simulink model "BaseEngineController_LS_112"  (Simulink 7.7)
settings: Solver=FixedStepDiscrete  StartTime=0.0  StopTime=10.0  RelTol=1e-3
PreLoadFcn:
  | try, eval([bdroot '_setup']); catch, eval('model_setup', ''); end
InitFcn:
  | try, eval([bdroot '_setup']); catch, eval('model_setup', ''); end
undefined symbols (not defined in the file): ECM, H1, H2, High, motohawk_build_version, motohawk_trunc_name, motohawk_vardec_config_group, motohawk_vardec_path, True, xD
libraries: MotoHawk_lib x1417, motohawk_control_primitives_lib x183, motohawk_engine_lib x32, simulink x21, motohawk_annotations_lib x9, AutoDoc_lib x8, simulink_extras x4, motohawk_ccp_examples_lib x1, motohawk_control_primitives_motoshare_lib x1
(part 10 of 27)

== system BaseEngineController_LS_112/Foreground/Outputs/AEM Infinity Dash/Dash Message Boost ==
  Data : Inport
  Bus Selector : BusSelector  OutputSignals=Sensors.Raw.NonLinearSensors.CAT
  Constant : Constant  Value=0
  Constant1 : Constant  Value=0
  Send CAN Messages : MotoHawk_lib/CAN Blocks/Send CAN Messages  bus=-2  nam='CAN_1'  msgl=CANTx_AEM_DASH_Boost  pace=5  labelwires=off
  motohawk_data_read : MotoHawk_lib/Data Storage Blocks/motohawk_data_read  source=Lookup By Name  structure=Scalar  operation=Read scalar from location by index  sz_vec=4  sz_row=2  sz_col=3  typ=double  nam='BoostControlTarget'  checkNull=on  struct_inst_name='MyData'  struct_nam='MyStruct'
  motohawk_data_read1 : MotoHawk_lib/Data Storage Blocks/motohawk_data_read  source=Lookup By Name  structure=Scalar  operation=Read scalar from location by index  sz_vec=4  sz_row=2  sz_col=3  typ=uint8  nam='BoostControlDutyCycleFF'  checkNull=on  struct_inst_name='MyData'  struct_nam='MyStruct'
  motohawk_data_read2 : MotoHawk_lib/Data Storage Blocks/motohawk_data_read  source=Lookup By Name  structure=Scalar  operation=Read scalar from location by index  sz_vec=4  sz_row=2  sz_col=3  typ=double  nam='BoostControlPID'  checkNull=on  struct_inst_name='MyData'  struct_nam='MyStruct'
  wires:
  Data/1 -> Bus Selector/1
  motohawk_data_read/1 -> Send CAN Messages/1
  Constant/1 -> Send CAN Messages/2
  motohawk_data_read1/1 -> Send CAN Messages/3
  motohawk_data_read2/1 -> Send CAN Messages/4
  Bus Selector/1 -> Send CAN Messages/5  "<CAT>"
  Constant1/1 -> Send CAN Messages/6

== system BaseEngineController_LS_112/Foreground/Outputs/AEM Infinity Dash/Dash Message DBW ==
  Data : Inport
  Bus Selector : BusSelector  OutputSignals=Sensors.RawProcessed.APPPcnt,Sensors.RawProcessed.ETCRequest,Sensors.Raw.PotSensors.TPS1,Sensors.Raw.PotSensors.TPS2
  Constant{1..8} (8 alike) : Constant  Value=0
  First Order Low Pass (Tunable) : motohawk_control_primitives_lib/First Order Low Pass (Tunable)  SystemSampleTime=-1  nam='ETCReq_Filt'  samp_time=-1  group=motohawk_vardec_path(gcb)
  First Order Low Pass (Tunable)1 : motohawk_control_primitives_lib/First Order Low Pass (Tunable)  SystemSampleTime=-1  nam='APP_Filt'  samp_time=-1  group=motohawk_vardec_path(gcb)
  Logical Operator{1..5} (5 alike) : Logic  Operator=OR  AllPortsSameDT=off  OutDataTypeStr=boolean
  Send CAN Messages : MotoHawk_lib/CAN Blocks/Send CAN Messages  bus=-2  nam='CAN_1'  msgl=CANTx_AEM_DASH_DBW  pace=5  labelwires=off
  motohawk_data_read1 : MotoHawk_lib/Data Storage Blocks/motohawk_data_read  source=Lookup By Name  structure=Scalar  operation=Read scalar from location by index  sz_vec=4  sz_row=2  sz_col=3  typ=boolean  nam='ETB_Curr_Flt'  checkNull=on  struct_inst_name='MyData'  struct_nam='MyStruct'
  motohawk_fault_status1 : MotoHawk_lib/Fault Management Blocks/motohawk_fault_status  source=Lookup By Name  nam='APP1RangeHigh'  status=Active
  motohawk_fault_status10 : MotoHawk_lib/Fault Management Blocks/motohawk_fault_status  source=Lookup By Name  nam='APP1RangeLow'  status=Active
  motohawk_fault_status11 : MotoHawk_lib/Fault Management Blocks/motohawk_fault_status  source=Lookup By Name  nam='TPS2RangeLow'  status=Active
  motohawk_fault_status12 : MotoHawk_lib/Fault Management Blocks/motohawk_fault_status  source=Lookup By Name  nam='TPS_Sensors_Conflict'  status=Active
  motohawk_fault_status2 : MotoHawk_lib/Fault Management Blocks/motohawk_fault_status  source=Lookup By Name  nam='APP2RangeHigh'  status=Active
  motohawk_fault_status3 : MotoHawk_lib/Fault Management Blocks/motohawk_fault_status  source=Lookup By Name  nam='APP2RangeLow'  status=Active
  motohawk_fault_status4 : MotoHawk_lib/Fault Management Blocks/motohawk_fault_status  source=Lookup By Name  nam='TPS1RangeHigh'  status=Active
  motohawk_fault_status5 : MotoHawk_lib/Fault Management Blocks/motohawk_fault_status  source=Lookup By Name  nam='ETC_Sticking'  status=Active
  motohawk_fault_status6 : MotoHawk_lib/Fault Management Blocks/motohawk_fault_status  source=Lookup By Name  nam='ETC_Open_Fault'  status=Active
  motohawk_fault_status7 : MotoHawk_lib/Fault Management Blocks/motohawk_fault_status  source=Lookup By Name  nam='TPS1RangeLow'  status=Active
  motohawk_fault_status8 : MotoHawk_lib/Fault Management Blocks/motohawk_fault_status  source=Lookup By Name  nam='TPS2RangeHigh'  status=Active
  motohawk_fault_status9 : MotoHawk_lib/Fault Management Blocks/motohawk_fault_status  source=Lookup By Name  nam='APP_Sensors_Conflict'  status=Active
  wires:
  Data/1 -> Bus Selector/1
  Bus Selector/1 -> First Order Low Pass (Tunable)1/1  "<APPPcnt>"
  Bus Selector/2 -> First Order Low Pass (Tunable)/1  "<ETCRequest>"
  Bus Selector/3 -> Send CAN Messages/3  "<TPS1>"
  Bus Selector/4 -> Send CAN Messages/4  "<TPS2>"
  motohawk_fault_status9/1 -> Send CAN Messages/5
  motohawk_fault_status10/1 -> Logical Operator3/1
  motohawk_fault_status1/1 -> Logical Operator3/2
  Logical Operator3/1 -> Send CAN Messages/6
  motohawk_fault_status3/1 -> Logical Operator1/1
  motohawk_fault_status2/1 -> Logical Operator1/2
  Logical Operator1/1 -> Send CAN Messages/7
  Constant1/1 -> Send CAN Messages/8
  Constant2/1 -> Send CAN Messages/20
  Constant3/1 -> Send CAN Messages/19
  Constant4/1 -> Send CAN Messages/18
  Constant5/1 -> Send CAN Messages/17
  Constant6/1 -> Send CAN Messages/16
  Constant7/1 -> Send CAN Messages/15
  motohawk_fault_status5/1 -> Logical Operator2/2
  motohawk_fault_status6/1 -> Logical Operator2/1
  Logical Operator2/1 -> Send CAN Messages/9
  motohawk_fault_status4/1 -> Logical Operator4/2
  motohawk_fault_status7/1 -> Logical Operator4/1
  Logical Operator4/1 -> Send CAN Messages/10
  motohawk_fault_status8/1 -> Logical Operator5/2
  motohawk_fault_status11/1 -> Logical Operator5/1
  Logical Operator5/1 -> Send CAN Messages/11
  motohawk_fault_status12/1 -> Send CAN Messages/14
  motohawk_data_read1/1 -> Send CAN Messages/13
  Constant8/1 -> Send CAN Messages/12
  First Order Low Pass (Tunable)1/1 -> Send CAN Messages/1
  First Order Low Pass (Tunable)/1 -> Send CAN Messages/2

== system BaseEngineController_LS_112/Foreground/Outputs/Coil Control/Coil Enable Manager ==
  CompareTo : motohawk_control_primitives_lib/CompareTo  SystemSampleTime=-1  op===  val=1
  EST Enable TDC Counter : Subsystem  TreatAsAtomicUnit=on
  Logical Operator1 : Logic  Operator=NOT  AllPortsSameDT=off  OutDataTypeStr=boolean
  Logical Operator2 : Logic  Inputs=6  AllPortsSameDT=off  OutDataTypeStr=boolean
  Logical Operator3 : Logic  Operator=NOT  AllPortsSameDT=off  OutDataTypeStr=boolean
  Logical Operator4 : Logic  Operator=NOT  AllPortsSameDT=off  OutDataTypeStr=boolean
  Mux : Mux  Inputs=8
  motohawk_calibration1 : MotoHawk_lib/Calibration & Probing Blocks/motohawk_calibration  nam='SparkEnableCyl5'  val=true  storage=Calibration  show_more=on  name_source=Use Parameter  data_type=Inherit via back propagation  read_level=1  write_level=1  ovr_cals=on  view_as=Enumeration  enum_struct={'Disabled', 'Enabled'}  vector_style=Wide Row  use_help_units=on  help='Disable spark to particular cylinder.'  units='boolean'  use_header_enum=off  row_header_enum={}  col_header_enum={}  use_min_max=off  min_val=-inf  max_val=inf  use_precision=off  precision=''  gain=1  offset=0  exp=1  use_mototune_group=on  mototune_group=motohawk_vardec_path(gcb)
  motohawk_calibration3 : MotoHawk_lib/Calibration & Probing Blocks/motohawk_calibration  nam='SparkEnableCyl1'  val=true  storage=Calibration  show_more=on  name_source=Use Parameter  data_type=Inherit via back propagation  read_level=1  write_level=1  ovr_cals=on  view_as=Enumeration  enum_struct={'Disabled', 'Enabled'}  vector_style=Wide Row  use_help_units=on  help='Disable spark to particular cylinder.'  units='boolean'  use_header_enum=off  row_header_enum={}  col_header_enum={}  use_min_max=off  min_val=-inf  max_val=inf  use_precision=off  precision=''  gain=1  offset=0  exp=1  use_mototune_group=on  mototune_group=motohawk_vardec_path(gcb)
  motohawk_calibration4 : MotoHawk_lib/Calibration & Probing Blocks/motohawk_calibration  nam='SparkEnableCyl2'  val=true  storage=Calibration  show_more=on  name_source=Use Parameter  data_type=Inherit via back propagation  read_level=1  write_level=1  ovr_cals=on  view_as=Enumeration  enum_struct={'Disabled', 'Enabled'}  vector_style=Wide Row  use_help_units=on  help='Disable spark to particular cylinder.'  units='boolean'  use_header_enum=off  row_header_enum={}  col_header_enum={}  use_min_max=off  min_val=-inf  max_val=inf  use_precision=off  precision=''  gain=1  offset=0  exp=1  use_mototune_group=on  mototune_group=motohawk_vardec_path(gcb)
  motohawk_calibration5 : MotoHawk_lib/Calibration & Probing Blocks/motohawk_calibration  nam='SparkEnableCyl3'  val=true  storage=Calibration  show_more=on  name_source=Use Parameter  data_type=Inherit via back propagation  read_level=1  write_level=1  ovr_cals=on  view_as=Enumeration  enum_struct={'Disabled', 'Enabled'}  vector_style=Wide Row  use_help_units=on  help='Disable spark to particular cylinder.'  units='boolean'  use_header_enum=off  row_header_enum={}  col_header_enum={}  use_min_max=off  min_val=-inf  max_val=inf  use_precision=off  precision=''  gain=1  offset=0  exp=1  use_mototune_group=on  mototune_group=motohawk_vardec_path(gcb)
  motohawk_calibration6 : MotoHawk_lib/Calibration & Probing Blocks/motohawk_calibration  nam='SparkEnableCyl4'  val=true  storage=Calibration  show_more=on  name_source=Use Parameter  data_type=Inherit via back propagation  read_level=1  write_level=1  ovr_cals=on  view_as=Enumeration  enum_struct={'Disabled', 'Enabled'}  vector_style=Wide Row  use_help_units=on  help='Disable spark to particular cylinder.'  units='boolean'  use_header_enum=off  row_header_enum={}  col_header_enum={}  use_min_max=off  min_val=-inf  max_val=inf  use_precision=off  precision=''  gain=1  offset=0  exp=1  use_mototune_group=on  mototune_group=motohawk_vardec_path(gcb)
  motohawk_calibration7 : MotoHawk_lib/Calibration & Probing Blocks/motohawk_calibration  nam='SparkEnableCyl6'  val=true  storage=Calibration  show_more=on  name_source=Use Parameter  data_type=Inherit via back propagation  read_level=1  write_level=1  ovr_cals=on  view_as=Enumeration  enum_struct={'Disabled', 'Enabled'}  vector_style=Wide Row  use_help_units=on  help='Disable spark to particular cylinder.'  units='boolean'  use_header_enum=off  row_header_enum={}  col_header_enum={}  use_min_max=off  min_val=-inf  max_val=inf  use_precision=off  precision=''  gain=1  offset=0  exp=1  use_mototune_group=on  mototune_group=motohawk_vardec_path(gcb)
  motohawk_calibration8 : MotoHawk_lib/Calibration & Probing Blocks/motohawk_calibration  nam='SparkEnableCyl7'  val=true  storage=Calibration  show_more=on  name_source=Use Parameter  data_type=Inherit via back propagation  read_level=1  write_level=1  ovr_cals=on  view_as=Enumeration  enum_struct={'Disabled', 'Enabled'}  vector_style=Wide Row  use_help_units=on  help='Disable spark to particular cylinder.'  units='boolean'  use_header_enum=off  row_header_enum={}  col_header_enum={}  use_min_max=off  min_val=-inf  max_val=inf  use_precision=off  precision=''  gain=1  offset=0  exp=1  use_mototune_group=on  mototune_group=motohawk_vardec_path(gcb)
  motohawk_calibration9 : MotoHawk_lib/Calibration & Probing Blocks/motohawk_calibration  nam='SparkEnableCyl8'  val=true  storage=Calibration  show_more=on  name_source=Use Parameter  data_type=Inherit via back propagation  read_level=1  write_level=1  ovr_cals=on  view_as=Enumeration  enum_struct={'Disabled', 'Enabled'}  vector_style=Wide Row  use_help_units=on  help='Disable spark to particular cylinder.'  units='boolean'  use_header_enum=off  row_header_enum={}  col_header_enum={}  use_min_max=off  min_val=-inf  max_val=inf  use_precision=off  precision=''  gain=1  offset=0  exp=1  use_mototune_group=on  mototune_group=motohawk_vardec_path(gcb)
  motohawk_data_def : MotoHawk_lib/Data Storage Blocks/motohawk_data_def  nam='EngineShutdownAction'  container_nam=''  data=0  typ=boolean  struct_nam='MyStruct'  storage=Volatile  outputRef=off  use_vardec=off  window=Calibration  read_level=1  write_level=1  ovr_cals=on  view_as=Number  enum_struct={'Disabled', 'Enabled'}  vector_style=Wide Row  use_help_units=on  help=''  units=''  use_header_enum=off  row_header_enum=''  col_header_enum=''  use_min_max=off  min_val=-inf  max_val=inf  use_precision=off  precision=''  gain=1  offset=0  exp=1  use_mototune_group=off  mototune_group=motohawk_vardec_path(gcb)  eval_name=EngineShutdownAction  data_stores=motohawk_sfun_data_def_data_stores  struct_instances=motohawk_sfun_data_def_struct_instances  vardecs=motohawk_sfun_data_def_vardecs
  motohawk_data_read1 : MotoHawk_lib/Data Storage Blocks/motohawk_data_read  source=Lookup By Name  structure=Scalar  operation=Read scalar from location by index  sz_vec=4  sz_row=2  sz_col=3  typ=boolean  nam='DelayedEngineShutdownAction'  checkNull=on  struct_inst_name='Struct1'  struct_nam='MyStruct'
  motohawk_data_read2 : MotoHawk_lib/Data Storage Blocks/motohawk_data_read  source=Lookup By Name  structure=Scalar  operation=Read scalar from location by index  sz_vec=4  sz_row=2  sz_col=3  typ=boolean  nam='ECUP_Enabled'  checkNull=on  struct_inst_name='Struct1'  struct_nam='MyStruct'
  motohawk_data_read3 : MotoHawk_lib/Data Storage Blocks/motohawk_data_read  source=Lookup By Name  structure=Scalar  operation=Read scalar from location by index  sz_vec=4  sz_row=2  sz_col=3  typ=uint8  nam='EngineState'  checkNull=on  struct_inst_name='Struct1'  struct_nam='MyStruct'
  motohawk_data_write : MotoHawk_lib/Data Storage Blocks/motohawk_data_write  source=Lookup By Name  structure=Scalar  operation=Write scalar into location by index  sz_vec=-1  sz_row=3  sz_col=2  typ=boolean  nam='EngineShutdownAction'  checkNull=on  write_read_only=off  struct_inst_name='Struct1'  struct_name='MyStruct'
  motohawk_fault_action : MotoHawk_lib/Fault Management Blocks/motohawk_fault_action  nam='EngineShutdown'  output_status=on  eval_nam=EngineShutdown
  Enable : Outport
  wires:
  EST Enable TDC Counter/1(Enable) -> Logical Operator2/6
  Logical Operator4/1 -> Logical Operator2/5
  CompareTo/1 -> Logical Operator4/1
  motohawk_data_read3/1 -> CompareTo/1
  Logical Operator3/1 -> Logical Operator2/1
  Logical Operator2/1 -> Enable/1
  motohawk_data_read2/1 -> Logical Operator2/4
  Mux/1 -> Logical Operator2/3
  Logical Operator1/1 -> Logical Operator2/2
  motohawk_calibration9/1 -> Mux/8
  motohawk_calibration8/1 -> Mux/7
  motohawk_calibration7/1 -> Mux/6
  motohawk_calibration1/1 -> Mux/5
  motohawk_data_read1/1 -> Logical Operator3/1
  motohawk_fault_action/1 -> Logical Operator1/1, motohawk_data_write/1
  motohawk_calibration6/1 -> Mux/4
  motohawk_calibration5/1 -> Mux/3
  motohawk_calibration4/1 -> Mux/2
  motohawk_calibration3/1 -> Mux/1

== system BaseEngineController_LS_112/Foreground/Outputs/Coil Control/EST Fault Management ==
  Short : Inport
  Open : Inport  Port=2
  OpenADC : Inport  Port=3
  Dwell : Inport  Port=4
  CompareTo{,1..15} (16 alike) : motohawk_control_primitives_lib/CompareTo  SystemSampleTime=-1  op===  val=1
  Demux : Demux  Outputs=8
  Demux1 : Demux  Outputs=8
  motohawk_fault_def : MotoHawk_lib/Fault Management Blocks/motohawk_fault_def  nam='EST1_Short'  mode=Enabled  id=[]  x=25  y=50  input_suspected=on  indeterminate=off  increment_xy=on  downsample_count=1  ovr_cals=on  ovr_actions=on  show_actions=off  action1_name=''  action1_cond=(None)  action2_name=''  action2_cond=(None)  action3_name=''  action3_cond=(None)  action4_name=''  action4_cond=(None)
  motohawk_fault_def1 : MotoHawk_lib/Fault Management Blocks/motohawk_fault_def  nam='EST2_Short'  mode=Enabled  id=[]  x=25  y=50  input_suspected=on  indeterminate=off  increment_xy=on  downsample_count=1  ovr_cals=on  ovr_actions=on  show_actions=off  action1_name=''  action1_cond=(None)  action2_name=''  action2_cond=(None)  action3_name=''  action3_cond=(None)  action4_name=''  action4_cond=(None)
  motohawk_fault_def10 : MotoHawk_lib/Fault Management Blocks/motohawk_fault_def  nam='EST3_Short'  mode=Enabled  id=[]  x=25  y=50  input_suspected=on  indeterminate=off  increment_xy=on  downsample_count=1  ovr_cals=on  ovr_actions=on  show_actions=off  action1_name=''  action1_cond=(None)  action2_name=''  action2_cond=(None)  action3_name=''  action3_cond=(None)  action4_name=''  action4_cond=(None)
  motohawk_fault_def11 : MotoHawk_lib/Fault Management Blocks/motohawk_fault_def  nam='EST4_Short'  mode=Enabled  id=[]  x=25  y=50  input_suspected=on  indeterminate=off  increment_xy=on  downsample_count=1  ovr_cals=on  ovr_actions=on  show_actions=off  action1_name=''  action1_cond=(None)  action2_name=''  action2_cond=(None)  action3_name=''  action3_cond=(None)  action4_name=''  action4_cond=(None)
  motohawk_fault_def12 : MotoHawk_lib/Fault Management Blocks/motohawk_fault_def  nam='EST5_Short'  mode=Enabled  id=[]  x=25  y=50  input_suspected=on  indeterminate=off  increment_xy=on  downsample_count=1  ovr_cals=on  ovr_actions=on  show_actions=off  action1_name=''  action1_cond=(None)  action2_name=''  action2_cond=(None)  action3_name=''  action3_cond=(None)  action4_name=''  action4_cond=(None)
  motohawk_fault_def13 : MotoHawk_lib/Fault Management Blocks/motohawk_fault_def  nam='EST6_Short'  mode=Enabled  id=[]  x=25  y=50  input_suspected=on  indeterminate=off  increment_xy=on  downsample_count=1  ovr_cals=on  ovr_actions=on  show_actions=off  action1_name=''  action1_cond=(None)  action2_name=''  action2_cond=(None)  action3_name=''  action3_cond=(None)  action4_name=''  action4_cond=(None)
  motohawk_fault_def14 : MotoHawk_lib/Fault Management Blocks/motohawk_fault_def  nam='EST7_Short'  mode=Enabled  id=[]  x=25  y=50  input_suspected=on  indeterminate=off  increment_xy=on  downsample_count=1  ovr_cals=on  ovr_actions=on  show_actions=off  action1_name=''  action1_cond=(None)  action2_name=''  action2_cond=(None)  action3_name=''  action3_cond=(None)  action4_name=''  action4_cond=(None)
  motohawk_fault_def15 : MotoHawk_lib/Fault Management Blocks/motohawk_fault_def  nam='EST8_Short'  mode=Enabled  id=[]  x=25  y=50  input_suspected=on  indeterminate=off  increment_xy=on  downsample_count=1  ovr_cals=on  ovr_actions=on  show_actions=off  action1_name=''  action1_cond=(None)  action2_name=''  action2_cond=(None)  action3_name=''  action3_cond=(None)  action4_name=''  action4_cond=(None)
  motohawk_fault_def2 : MotoHawk_lib/Fault Management Blocks/motohawk_fault_def  nam='EST3_Open'  mode=Enabled  id=[]  x=25  y=50  input_suspected=on  indeterminate=off  increment_xy=on  downsample_count=1  ovr_cals=on  ovr_actions=on  show_actions=off  action1_name=''  action1_cond=(None)  action2_name=''  action2_cond=(None)  action3_name=''  action3_cond=(None)  action4_name=''  action4_cond=(None)
  motohawk_fault_def3 : MotoHawk_lib/Fault Management Blocks/motohawk_fault_def  nam='EST4_Open'  mode=Enabled  id=[]  x=25  y=50  input_suspected=on  indeterminate=off  increment_xy=on  downsample_count=1  ovr_cals=on  ovr_actions=on  show_actions=off  action1_name=''  action1_cond=(None)  action2_name=''  action2_cond=(None)  action3_name=''  action3_cond=(None)  action4_name=''  action4_cond=(None)
  motohawk_fault_def4 : MotoHawk_lib/Fault Management Blocks/motohawk_fault_def  nam='EST5_Open'  mode=Enabled  id=[]  x=25  y=50  input_suspected=on  indeterminate=off  increment_xy=on  downsample_count=1  ovr_cals=on  ovr_actions=on  show_actions=off  action1_name=''  action1_cond=(None)  action2_name=''  action2_cond=(None)  action3_name=''  action3_cond=(None)  action4_name=''  action4_cond=(None)
  motohawk_fault_def5 : MotoHawk_lib/Fault Management Blocks/motohawk_fault_def  nam='EST6_Open'  mode=Enabled  id=[]  x=25  y=50  input_suspected=on  indeterminate=off  increment_xy=on  downsample_count=1  ovr_cals=on  ovr_actions=on  show_actions=off  action1_name=''  action1_cond=(None)  action2_name=''  action2_cond=(None)  action3_name=''  action3_cond=(None)  action4_name=''  action4_cond=(None)
  motohawk_fault_def6 : MotoHawk_lib/Fault Management Blocks/motohawk_fault_def  nam='EST7_Open'  mode=Enabled  id=[]  x=25  y=50  input_suspected=on  indeterminate=off  increment_xy=on  downsample_count=1  ovr_cals=on  ovr_actions=on  show_actions=off  action1_name=''  action1_cond=(None)  action2_name=''  action2_cond=(None)  action3_name=''  action3_cond=(None)  action4_name=''  action4_cond=(None)
  motohawk_fault_def7 : MotoHawk_lib/Fault Management Blocks/motohawk_fault_def  nam='EST8_Open'  mode=Enabled  id=[]  x=25  y=50  input_suspected=on  indeterminate=off  increment_xy=on  downsample_count=1  ovr_cals=on  ovr_actions=on  show_actions=off  action1_name=''  action1_cond=(None)  action2_name=''  action2_cond=(None)  action3_name=''  action3_cond=(None)  action4_name=''  action4_cond=(None)
  motohawk_fault_def8 : MotoHawk_lib/Fault Management Blocks/motohawk_fault_def  nam='EST1_Open'  mode=Enabled  id=[]  x=25  y=50  input_suspected=on  indeterminate=off  increment_xy=on  downsample_count=1  ovr_cals=on  ovr_actions=on  show_actions=off  action1_name=''  action1_cond=(None)  action2_name=''  action2_cond=(None)  action3_name=''  action3_cond=(None)  action4_name=''  action4_cond=(None)
  motohawk_fault_def9 : MotoHawk_lib/Fault Management Blocks/motohawk_fault_def  nam='EST2_Open'  mode=Enabled  id=[]  x=25  y=50  input_suspected=on  indeterminate=off  increment_xy=on  downsample_count=1  ovr_cals=on  ovr_actions=on  show_actions=off  action1_name=''  action1_cond=(None)  action2_name=''  action2_cond=(None)  action3_name=''  action3_cond=(None)  action4_name=''  action4_cond=(None)
  motohawk_probe1 : MotoHawk_lib/Calibration & Probing Blocks/motohawk_probe  nam='EST_DiagDwell'  show_more=on  name_source=Use Parameter  read_level=1  view_as=Number  enum_struct={'Disabled', 'Enabled'}  vector_style=Wide Row  use_help_units=on  help='Dwell time used to diagnose ESTs during run-state.'  units='us'  use_header_enum=off  row_header_enum={}  col_header_enum={}  use_precision=off  precision=''  gain=1  offset=0  exp=1  use_mototune_group=on  mototune_group=motohawk_vardec_path(gcb)
  motohawk_probe5 : MotoHawk_lib/Calibration & Probing Blocks/motohawk_probe  nam='ESTOpenADC'  show_more=on  name_source=Use Parameter  read_level=1  view_as=Number  enum_struct={'Disabled', 'Enabled'}  vector_style=Wide Row  use_help_units=on  help='ADC counts of measured voltage feedback for diagnosing the ESTs during stall state.'  units=''  use_header_enum=off  row_header_enum={}  col_header_enum={}  use_precision=off  precision=''  gain=1  offset=0  exp=1  use_mototune_group=on  mototune_group=motohawk_vardec_path(gcb)
  wires:
  CompareTo9/1 -> motohawk_fault_def1/1
  CompareTo8/1 -> motohawk_fault_def/1
  CompareTo1/1 -> motohawk_fault_def9/1
  CompareTo/1 -> motohawk_fault_def8/1
  Dwell/1 -> motohawk_probe1/1
  Short/1 -> Demux1/1
  Demux1/2 -> CompareTo9/1
  Demux1/1 -> CompareTo8/1
  Open/1 -> Demux/1
  Demux/2 -> CompareTo1/1
  Demux/1 -> CompareTo/1
  OpenADC/1 -> motohawk_probe5/1
  CompareTo2/1 -> motohawk_fault_def2/1
  Demux/3 -> CompareTo2/1
  CompareTo3/1 -> motohawk_fault_def3/1
  Demux/4 -> CompareTo3/1
  CompareTo4/1 -> motohawk_fault_def4/1
  Demux/5 -> CompareTo4/1
  CompareTo5/1 -> motohawk_fault_def5/1
  Demux/6 -> CompareTo5/1
  CompareTo6/1 -> motohawk_fault_def6/1
  Demux/7 -> CompareTo6/1
  CompareTo7/1 -> motohawk_fault_def7/1
  Demux/8 -> CompareTo7/1
  CompareTo10/1 -> motohawk_fault_def10/1
  Demux1/3 -> CompareTo10/1
  CompareTo11/1 -> motohawk_fault_def11/1
  Demux1/4 -> CompareTo11/1
  CompareTo12/1 -> motohawk_fault_def12/1
  Demux1/5 -> CompareTo12/1
  CompareTo13/1 -> motohawk_fault_def13/1
  Demux1/6 -> CompareTo13/1
  CompareTo14/1 -> motohawk_fault_def14/1
  Demux1/7 -> CompareTo14/1
  CompareTo15/1 -> motohawk_fault_def15/1
  Demux1/8 -> CompareTo15/1

== system BaseEngineController_LS_112/Foreground/Outputs/Injector Control/Injector Diagnostics ==
  note: Non-Zero RPM
  Inj_Enabled : Inport
  TX Count : Inport  Port=2
  <1 : RelationalOperator  Operator=>  ZeroCross=off  InputSameDT=on
  == : RelationalOperator  Operator===  ZeroCross=off  InputSameDT=on
  AND1 : Logic  Inputs=3
  Demux : Demux  Outputs=8
  Zero : Constant  Value=0  OutDataTypeStr=uint8
  Zero1 : Constant  Value=100  OutDataTypeStr=Inherit: Inherit via back propagation
  motohawk_encoder_average_rpm : MotoHawk_lib/Encoder Blocks/motohawk_encoder_average_rpm
  motohawk_fault_def : MotoHawk_lib/Fault Management Blocks/motohawk_fault_def  nam='Inj1Open'  mode=Enabled  id=[]  x=25  y=50  input_suspected=on  indeterminate=off  increment_xy=on  downsample_count=1  ovr_cals=on  ovr_actions=on  show_actions=off  action1_name=''  action1_cond=(None)  action2_name=''  action2_cond=(None)  action3_name=''  action3_cond=(None)  action4_name=''  action4_cond=(None)
  motohawk_fault_def1 : MotoHawk_lib/Fault Management Blocks/motohawk_fault_def  nam='Inj2Open'  mode=Enabled  id=[]  x=25  y=50  input_suspected=on  indeterminate=off  increment_xy=on  downsample_count=1  ovr_cals=on  ovr_actions=on  show_actions=off  action1_name=''  action1_cond=(None)  action2_name=''  action2_cond=(None)  action3_name=''  action3_cond=(None)  action4_name=''  action4_cond=(None)
  motohawk_fault_def2 : MotoHawk_lib/Fault Management Blocks/motohawk_fault_def  nam='Inj3Open'  mode=Enabled  id=[]  x=25  y=50  input_suspected=on  indeterminate=off  increment_xy=on  downsample_count=1  ovr_cals=on  ovr_actions=on  show_actions=off  action1_name=''  action1_cond=(None)  action2_name=''  action2_cond=(None)  action3_name=''  action3_cond=(None)  action4_name=''  action4_cond=(None)
  motohawk_fault_def3 : MotoHawk_lib/Fault Management Blocks/motohawk_fault_def  nam='Inj4Open'  mode=Enabled  id=[]  x=25  y=50  input_suspected=on  indeterminate=off  increment_xy=on  downsample_count=1  ovr_cals=on  ovr_actions=on  show_actions=off  action1_name=''  action1_cond=(None)  action2_name=''  action2_cond=(None)  action3_name=''  action3_cond=(None)  action4_name=''  action4_cond=(None)
  motohawk_fault_def4 : MotoHawk_lib/Fault Management Blocks/motohawk_fault_def  nam='Inj5Open'  mode=Enabled  id=[]  x=25  y=50  input_suspected=on  indeterminate=off  increment_xy=on  downsample_count=1  ovr_cals=on  ovr_actions=on  show_actions=off  action1_name=''  action1_cond=(None)  action2_name=''  action2_cond=(None)  action3_name=''  action3_cond=(None)  action4_name=''  action4_cond=(None)
  motohawk_fault_def5 : MotoHawk_lib/Fault Management Blocks/motohawk_fault_def  nam='Inj6Open'  mode=Enabled  id=[]  x=25  y=50  input_suspected=on  indeterminate=off  increment_xy=on  downsample_count=1  ovr_cals=on  ovr_actions=on  show_actions=off  action1_name=''  action1_cond=(None)  action2_name=''  action2_cond=(None)  action3_name=''  action3_cond=(None)  action4_name=''  action4_cond=(None)
  motohawk_fault_def6 : MotoHawk_lib/Fault Management Blocks/motohawk_fault_def  nam='Inj7Open'  mode=Enabled  id=[]  x=25  y=50  input_suspected=on  indeterminate=off  increment_xy=on  downsample_count=1  ovr_cals=on  ovr_actions=on  show_actions=off  action1_name=''  action1_cond=(None)  action2_name=''  action2_cond=(None)  action3_name=''  action3_cond=(None)  action4_name=''  action4_cond=(None)
  motohawk_fault_def7 : MotoHawk_lib/Fault Management Blocks/motohawk_fault_def  nam='Inj8Open'  mode=Enabled  id=[]  x=25  y=50  input_suspected=on  indeterminate=off  increment_xy=on  downsample_count=1  ovr_cals=on  ovr_actions=on  show_actions=off  action1_name=''  action1_cond=(None)  action2_name=''  action2_cond=(None)  action3_name=''  action3_cond=(None)  action4_name=''  action4_cond=(None)
  motohawk_probe : MotoHawk_lib/Calibration & Probing Blocks/motohawk_probe  nam=[prefix 'TransitionCount']  show_more=on  name_source=Use Parameter  read_level=1  view_as=Number  enum_struct={'Disabled', 'Enabled'}  vector_style=Wide Row  use_help_units=off  help=''  units=''  use_header_enum=off  row_header_enum={}  col_header_enum={}  use_precision=off  precision=''  gain=1  offset=0  exp=1  use_mototune_group=on  mototune_group=group
  wires:
  Inj_Enabled/1 -> AND1/3
  Demux/2 -> motohawk_fault_def1/1
  Demux/1 -> motohawk_fault_def/1
  <1/1 -> AND1/2
  AND1/1 -> Demux/1
  Zero1/1 -> <1/2
  motohawk_encoder_average_rpm/1 -> <1/1
  TX Count/1 -> motohawk_probe/1, ==/1
  ==/1 -> AND1/1
  Zero/1 -> ==/2
  Demux/3 -> motohawk_fault_def2/1
  Demux/4 -> motohawk_fault_def3/1
  Demux/5 -> motohawk_fault_def4/1
  Demux/6 -> motohawk_fault_def5/1
  Demux/7 -> motohawk_fault_def6/1
  Demux/8 -> motohawk_fault_def7/1

== system BaseEngineController_LS_112/Foreground/Outputs/Injector Control/Injector Enable Manager ==
  Constant : Constant  Value=0
  Constant1 : Constant  Value=true
  Gain : Gain  Gain=.5
  Logical Operator : Logic  Operator=NOT  AllPortsSameDT=off  OutDataTypeStr=boolean
  Logical Operator1 : Logic  Inputs=6  AllPortsSameDT=off  OutDataTypeStr=boolean
  Logical Operator2 : Logic  Operator=NOT  AllPortsSameDT=off  OutDataTypeStr=boolean
  Logical Operator4 : Logic  Operator=NOT  AllPortsSameDT=off  OutDataTypeStr=boolean
  Mux : Mux  Inputs=8
  Relational Operator : RelationalOperator  Operator=>  InputSameDT=on
  Relational Operator1 : RelationalOperator  Operator=>  InputSameDT=on
  Relational Operator2 : RelationalOperator  Operator=>  InputSameDT=on
  Stall : motohawk_control_primitives_lib/CompareTo  SystemSampleTime=-1  op===  val=1
  Time Since Enabled (With Input)1 : motohawk_control_primitives_lib/Time Since Enabled (With Input)1  SystemSampleTime=-1  nam='DelayedEngineShutdownTimer'  samp_time=.005  init=0  upperlim=16000
  motohawk_calibration1 : MotoHawk_lib/Calibration & Probing Blocks/motohawk_calibration  nam='EngineShutdownDelayTime'  val=20  storage=Calibration  show_more=on  name_source=Use Parameter  data_type=Inherit from 'Default Value'  read_level=1  write_level=1  ovr_cals=on  view_as=Number  enum_struct={'Disabled', 'Enabled'}  vector_style=Wide Row  use_help_units=on  help='Delays the engine shutdown when DelayedEngineShutdown fault-action is active.'  units='s'  use_header_enum=off  row_header_enum={}  col_header_enum={}  use_min_max=on  min_val=0  max_val=inf  use_precision=off  precision=''  gain=1  offset=0  exp=1  use_mototune_group=on  mototune_group=motohawk_vardec_path(gcb)
  motohawk_calibration10 : MotoHawk_lib/Calibration & Probing Blocks/motohawk_calibration  nam='Injector6Enable'  val=true  storage=Calibration  show_more=on  name_source=Use Parameter  data_type=Inherit from 'Default Value'  read_level=1  write_level=1  ovr_cals=on  view_as=Enumeration  enum_struct={'Disabled', 'Enabled'}  vector_style=Wide Row  use_help_units=off  help=''  units=''  use_header_enum=off  row_header_enum={}  col_header_enum={}  use_min_max=off  min_val=-inf  max_val=inf  use_precision=off  precision=''  gain=1  offset=0  exp=1  use_mototune_group=on  mototune_group=motohawk_vardec_path(gcb)
  motohawk_calibration11 : MotoHawk_lib/Calibration & Probing Blocks/motohawk_calibration  nam='Injector7Enable'  val=true  storage=Calibration  show_more=on  name_source=Use Parameter  data_type=Inherit from 'Default Value'  read_level=1  write_level=1  ovr_cals=on  view_as=Enumeration  enum_struct={'Disabled', 'Enabled'}  vector_style=Wide Row  use_help_units=off  help=''  units=''  use_header_enum=off  row_header_enum={}  col_header_enum={}  use_min_max=off  min_val=-inf  max_val=inf  use_precision=off  precision=''  gain=1  offset=0  exp=1  use_mototune_group=on  mototune_group=motohawk_vardec_path(gcb)
  motohawk_calibration12 : MotoHawk_lib/Calibration & Probing Blocks/motohawk_calibration  nam='Injector8Enable'  val=true  storage=Calibration  show_more=on  name_source=Use Parameter  data_type=Inherit from 'Default Value'  read_level=1  write_level=1  ovr_cals=on  view_as=Enumeration  enum_struct={'Disabled', 'Enabled'}  vector_style=Wide Row  use_help_units=off  help=''  units=''  use_header_enum=off  row_header_enum={}  col_header_enum={}  use_min_max=off  min_val=-inf  max_val=inf  use_precision=off  precision=''  gain=1  offset=0  exp=1  use_mototune_group=on  mototune_group=motohawk_vardec_path(gcb)
  motohawk_calibration2 : MotoHawk_lib/Calibration & Probing Blocks/motohawk_calibration  nam='Injector2Enable'  val=true  storage=Calibration  show_more=on  name_source=Use Parameter  data_type=Inherit from 'Default Value'  read_level=1  write_level=1  ovr_cals=on  view_as=Enumeration  enum_struct={'Disabled', 'Enabled'}  vector_style=Wide Row  use_help_units=off  help=''  units=''  use_header_enum=off  row_header_enum={}  col_header_enum={}  use_min_max=off  min_val=-inf  max_val=inf  use_precision=off  precision=''  gain=1  offset=0  exp=1  use_mototune_group=on  mototune_group=motohawk_vardec_path(gcb)
  motohawk_calibration3 : MotoHawk_lib/Calibration & Probing Blocks/motohawk_calibration  nam='Injector5Enable'  val=true  storage=Calibration  show_more=on  name_source=Use Parameter  data_type=Inherit from 'Default Value'  read_level=1  write_level=1  ovr_cals=on  view_as=Enumeration  enum_struct={'Disabled', 'Enabled'}  vector_style=Wide Row  use_help_units=off  help=''  units=''  use_header_enum=off  row_header_enum={}  col_header_enum={}  use_min_max=off  min_val=-inf  max_val=inf  use_precision=off  precision=''  gain=1  offset=0  exp=1  use_mototune_group=on  mototune_group=motohawk_vardec_path(gcb)
  motohawk_calibration4 : MotoHawk_lib/Calibration & Probing Blocks/motohawk_calibration  nam='Injector3Enable'  val=true  storage=Calibration  show_more=on  name_source=Use Parameter  data_type=Inherit from 'Default Value'  read_level=1  write_level=1  ovr_cals=on  view_as=Enumeration  enum_struct={'Disabled', 'Enabled'}  vector_style=Wide Row  use_help_units=off  help=''  units=''  use_header_enum=off  row_header_enum={}  col_header_enum={}  use_min_max=off  min_val=-inf  max_val=inf  use_precision=off  precision=''  gain=1  offset=0  exp=1  use_mototune_group=on  mototune_group=motohawk_vardec_path(gcb)
  motohawk_calibration7 : MotoHawk_lib/Calibration & Probing Blocks/motohawk_calibration  nam='Injector1Enable'  val=true  storage=Calibration  show_more=on  name_source=Use Parameter  data_type=Inherit from 'Default Value'  read_level=1  write_level=1  ovr_cals=on  view_as=Enumeration  enum_struct={'Disabled', 'Enabled'}  vector_style=Wide Row  use_help_units=off  help=''  units=''  use_header_enum=off  row_header_enum={}  col_header_enum={}  use_min_max=off  min_val=-inf  max_val=inf  use_precision=off  precision=''  gain=1  offset=0  exp=1  use_mototune_group=on  mototune_group=motohawk_vardec_path(gcb)
  motohawk_calibration8 : MotoHawk_lib/Calibration & Probing Blocks/motohawk_calibration  nam='Injector4Enable'  val=true  storage=Calibration  show_more=on  name_source=Use Parameter  data_type=Inherit from 'Default Value'  read_level=1  write_level=1  ovr_cals=on  view_as=Enumeration  enum_struct={'Disabled', 'Enabled'}  vector_style=Wide Row  use_help_units=off  help=''  units=''  use_header_enum=off  row_header_enum={}  col_header_enum={}  use_min_max=off  min_val=-inf  max_val=inf  use_precision=off  precision=''  gain=1  offset=0  exp=1  use_mototune_group=on  mototune_group=motohawk_vardec_path(gcb)
  motohawk_data_def : MotoHawk_lib/Data Storage Blocks/motohawk_data_def  nam='DelayedEngineShutdownAction'  container_nam=''  data=0  typ=boolean  struct_nam='MyStruct'  storage=Volatile  outputRef=off  use_vardec=off  window=Calibration  read_level=1  write_level=1  ovr_cals=on  view_as=Number  enum_struct={'Disabled', 'Enabled'}  vector_style=Wide Row  use_help_units=off  help=''  units=''  use_header_enum=off  row_header_enum={}  col_header_enum={}  use_min_max=off  min_val=-inf  max_val=inf  use_precision=off  precision=''  gain=1  offset=0  exp=1  use_mototune_group=off  mototune_group=motohawk_vardec_path(gcb)  eval_name=DelayedEngineShutdownAction  data_stores=motohawk_sfun_data_def_data_stores  struct_instances=motohawk_sfun_data_def_struct_instances  vardecs=motohawk_sfun_data_def_vardecs
  motohawk_data_def1 : MotoHawk_lib/Data Storage Blocks/motohawk_data_def  nam='DelayedEngineShutdownWarning'  container_nam=''  data=0  typ=boolean  struct_nam='MyStruct'  storage=Volatile  outputRef=off  use_vardec=off  window=Calibration  read_level=1  write_level=1  ovr_cals=on  view_as=Number  enum_struct={'Disabled', 'Enabled'}  vector_style=Wide Row  use_help_units=off  help=''  units=''  use_header_enum=off  row_header_enum={}  col_header_enum={}  use_min_max=off  min_val=-inf  max_val=inf  use_precision=off  precision=''  gain=1  offset=0  exp=1  use_mototune_group=off  mototune_group=motohawk_vardec_path(gcb)  eval_name=DelayedEngineShutdownWarning  data_stores=motohawk_sfun_data_def_data_stores  struct_instances=motohawk_sfun_data_def_struct_instances  vardecs=motohawk_sfun_data_def_vardecs
  motohawk_data_def2 : MotoHawk_lib/Data Storage Blocks/motohawk_data_def  nam='EngineShutdownTimerState'  container_nam=''  data=0  typ=boolean  struct_nam='MyStruct'  storage=Volatile  outputRef=off  use_vardec=off  window=Calibration  read_level=1  write_level=1  ovr_cals=on  view_as=Number  enum_struct={'Disabled', 'Enabled'}  vector_style=Wide Row  use_help_units=off  help=''  units=''  use_header_enum=off  row_header_enum={}  col_header_enum={}  use_min_max=off  min_val=-inf  max_val=inf  use_precision=off  precision=''  gain=1  offset=0  exp=1  use_mototune_group=off  mototune_group=motohawk_vardec_path(gcb)  eval_name=EngineShutdownTimerState  data_stores=motohawk_sfun_data_def_data_stores  struct_instances=motohawk_sfun_data_def_struct_instances  vardecs=motohawk_sfun_data_def_vardecs
  motohawk_data_read : MotoHawk_lib/Data Storage Blocks/motohawk_data_read  source=Lookup By Name  structure=Scalar  operation=Read scalar from location by index  sz_vec=4  sz_row=2  sz_col=3  typ=boolean  nam='EngineShutdownAction'  checkNull=on  struct_inst_name='Struct1'  struct_nam='MyStruct'
  motohawk_data_read1 : MotoHawk_lib/Data Storage Blocks/motohawk_data_read  source=Lookup By Name  structure=Scalar  operation=Read scalar from location by index  sz_vec=4  sz_row=2  sz_col=3  typ=boolean  nam='ECUP_Enabled'  checkNull=on  struct_inst_name='Struct1'  struct_nam='MyStruct'
  motohawk_data_read2 : MotoHawk_lib/Data Storage Blocks/motohawk_data_read  source=Lookup By Name  structure=Scalar  operation=Read scalar from location by index  sz_vec=4  sz_row=2  sz_col=3  typ=uint8  nam='EngineState'  checkNull=on  struct_inst_name='Struct1'  struct_nam='MyStruct'
  motohawk_data_write : MotoHawk_lib/Data Storage Blocks/motohawk_data_write  source=Lookup By Name  structure=Scalar  operation=Write scalar into location by index  sz_vec=-1  sz_row=3  sz_col=2  typ=boolean  nam='DelayedEngineShutdownAction'  checkNull=on  write_read_only=off  struct_inst_name='Struct1'  struct_name='MyStruct'
  motohawk_data_write1 : MotoHawk_lib/Data Storage Blocks/motohawk_data_write  source=Lookup By Name  structure=Scalar  operation=Write scalar into location by index  sz_vec=-1  sz_row=3  sz_col=2  typ=boolean  nam='DelayedEngineShutdownWarning'  checkNull=on  write_read_only=off  struct_inst_name='Struct1'  struct_name='MyStruct'
  motohawk_data_write2 : MotoHawk_lib/Data Storage Blocks/motohawk_data_write  source=Lookup By Name  structure=Scalar  operation=Write scalar into location by index  sz_vec=-1  sz_row=3  sz_col=2  typ=boolean  nam='EngineShutdownTimerState'  checkNull=on  write_read_only=off  struct_inst_name='Struct1'  struct_name='MyStruct'
  motohawk_fault_action : MotoHawk_lib/Fault Management Blocks/motohawk_fault_action  nam='DelayedEngineShutdown'  output_status=on  eval_nam=DelayedEngineShutdown
  Enable : Outport
  wires:
  Relational Operator2/1 -> motohawk_data_write2/1
  Constant/1 -> Relational Operator2/2
  Relational Operator1/1 -> motohawk_data_write1/1
  Gain/1 -> Relational Operator1/2
  motohawk_fault_action/1 -> Time Since Enabled (With Input)1/1
  Mux/1 -> Logical Operator1/6
  motohawk_calibration12/1 -> Mux/8
  motohawk_calibration11/1 -> Mux/7
  motohawk_calibration10/1 -> Mux/6
  motohawk_calibration3/1 -> Mux/5
  motohawk_calibration8/1 -> Mux/4
  motohawk_calibration4/1 -> Mux/3
  motohawk_calibration2/1 -> Mux/2
  motohawk_calibration7/1 -> Mux/1
  Logical Operator4/1 -> Logical Operator1/5
  Stall/1 -> Logical Operator4/1
  motohawk_data_read2/1 -> Stall/1
  motohawk_calibration1/1 -> Gain/1, Relational Operator/2
  Time Since Enabled (With Input)1/1 -> Relational Operator2/1, Relational Operator1/1, Relational Operator/1
  Relational Operator/1 -> Logical Operator/1, motohawk_data_write/1
  Logical Operator/1 -> Logical Operator1/1
  Logical Operator1/1 -> Enable/1
  motohawk_data_read/1 -> Logical Operator2/1
  Logical Operator2/1 -> Logical Operator1/2
  Constant1/1 -> Logical Operator1/3
  motohawk_data_read1/1 -> Logical Operator1/4

== system BaseEngineController_LS_112/Main Power Relay/Main Power Relay/Forced Shutdown Process/Post Shutdown two ticks before MPRD off ==
  Trigger : TriggerPort  TriggerType=falling
  Constant : Constant  Value=true
  Function-Call Generator : simulink/Ports & Subsystems/Function-Call Generator  sample_time=-1  numberOfIterations=1
  Post Shutdown two ticks before MPRD off : MotoHawk_lib/Trigger Blocks/motohawk_event_call  SystemSampleTime=-1  mode=Post Event  trigger=SHUTDOWN_EVENT  target=ECM_5554_112_0904_xD
  motohawk_code_coverage : MotoHawk_lib/Extra Development Blocks/motohawk_code_coverage
  motohawk_single_fault_clear : MotoHawk_lib/Fault Management Blocks/motohawk_single_fault_clear  source=Lookup By Name  nam='ETCSpringTest'
  wires:
  Constant/1 -> motohawk_single_fault_clear/1
  Function-Call Generator/1 -> Post Shutdown two ticks before MPRD off/Trigger

== system BaseEngineController_LS_112/Main Power Relay/Main Power Relay/Forced Shutdown Process/Processor Reboot ==
  Trigger : TriggerPort  TriggerType=falling
  Loop Forever Causing Watchdog Reset : MotoHawk_lib/Extra Development Blocks/motohawk_inline_code  include_code=''  start_code=''  output_code='while (1);'
  motohawk_code_coverage : MotoHawk_lib/Extra Development Blocks/motohawk_code_coverage

== system BaseEngineController_LS_112/Main Power Relay/Main Power Relay/Forced Shutdown Process/Save NV Vars one tick before MPRD off ==
  Trigger : TriggerPort  TriggerType=falling
  Function-Call Generator : simulink/Ports & Subsystems/Function-Call Generator  sample_time=-1  numberOfIterations=1
  Save NV Vars one tick before MPRD off : MotoHawk_lib/Data Storage Blocks/motohawk_store_nvmem  SystemSampleTime=-1
  motohawk_code_coverage : MotoHawk_lib/Extra Development Blocks/motohawk_code_coverage
  wires:
  Function-Call Generator/1 -> Save NV Vars one tick before MPRD off/Trigger

== system BaseEngineController_LS_112/Main Power Relay/Main Power Relay/Forced Shutdown Process/Shutdown power on ECU565/563 ==
  Trigger : TriggerPort  TriggerType=falling
  Function-Call Generator : simulink/Ports & Subsystems/Function-Call Generator  sample_time=-1  numberOfIterations=1
  Shutdown power on ECU565-128 : MotoHawk_lib/Extra Development Blocks/motohawk_shutdown_power  SystemSampleTime=-1
  motohawk_code_coverage : MotoHawk_lib/Extra Development Blocks/motohawk_code_coverage
  wires:
  Function-Call Generator/1 -> Shutdown power on ECU565-128/Trigger

== system BaseEngineController_LS_112/Main Power Relay/Main Power Relay/ShutDown Processes/Post Shutdown two ticks before MPRD off ==
  Trigger : TriggerPort  TriggerType=falling
  Function-Call Generator : simulink/Ports & Subsystems/Function-Call Generator  sample_time=-1  numberOfIterations=1
  Post Shutdown two ticks before MPRD off : MotoHawk_lib/Trigger Blocks/motohawk_event_call  SystemSampleTime=-1  mode=Post Event  trigger=SHUTDOWN_EVENT  target=ECM_5554_112_0904_xD
  wires:
  Function-Call Generator/1 -> Post Shutdown two ticks before MPRD off/Trigger

== system BaseEngineController_LS_112/Main Power Relay/Main Power Relay/ShutDown Processes/Processor Reboot ==
  Enable : EnablePort
  Trigger : TriggerPort  TriggerType=falling
  Loop Forever Causing Watchdog Reset : MotoHawk_lib/Extra Development Blocks/motohawk_inline_code  include_code=''  start_code=''  output_code='while (1);'

== system BaseEngineController_LS_112/Main Power Relay/Main Power Relay/ShutDown Processes/Save NV Vars one tick before MPRD off ==
  Trigger : TriggerPort  TriggerType=falling
  Function-Call Generator1 : simulink/Ports & Subsystems/Function-Call Generator  sample_time=-1  numberOfIterations=1
  Save NV Vars one tick before MPRD off : MotoHawk_lib/Data Storage Blocks/motohawk_store_nvmem  SystemSampleTime=-1
  wires:
  Function-Call Generator1/1 -> Save NV Vars one tick before MPRD off/Trigger

== system BaseEngineController_LS_112/Main Power Relay/Main Power Relay/ShutDown Processes/Shutdown power on ECU565/563 ==
  Trigger : TriggerPort  TriggerType=falling
  Function-Call Generator2 : simulink/Ports & Subsystems/Function-Call Generator  sample_time=-1  numberOfIterations=1
  Shutdown power on ECU565-128 : MotoHawk_lib/Extra Development Blocks/motohawk_shutdown_power  SystemSampleTime=-1
  wires:
  Function-Call Generator2/1 -> Shutdown power on ECU565-128/Trigger

== system BaseEngineController_LS_112/Foreground/Control/ActuatorCharacterization/Electronic Throttle Controller/ETC Adapt Request ==
  ETC Setpoint Mode : Inport
  ETC Error : Inport  Port=2
  Add1 : Sum
  Constant1 : Constant  Value=5  SampleTime=-1
  Documentation_Calibrations_Probes_Block : AutoDoc_lib/Documentation_Calibrations_Probes_Block
  Logical Operator : Logic  AllPortsSameDT=off  OutDataTypeStr=boolean
  Relational Operator4 : RelationalOperator  Operator=<=  ZeroCross=off  InputSameDT=on
  ShutDownAdaptMode : motohawk_control_primitives_lib/CompareTo  SystemSampleTime=-1  op===  val=1
  motohawk_data_def1 : MotoHawk_lib/Data Storage Blocks/motohawk_data_def  nam='TPSAdaptLoRequest'  container_nam=''  data=false  typ=Inherit from 'Initial Value'  struct_nam='MyStruct'  storage=Volatile  outputRef=off  use_vardec=off  window=Display  read_level=1  write_level=1  ovr_cals=on  view_as=Number  enum_struct={'Disabled', 'Enabled'}  vector_style=Wide Row  use_help_units=off  help=''  units=''  use_header_enum=off  row_header_enum={}  col_header_enum={}  use_min_max=off  min_val=-inf  max_val=inf  use_precision=off  precision=''  gain=1  offset=0  exp=1  use_mototune_group=on  mototune_group=motohawk_vardec_path(gcb)  eval_name=TPSAdaptLoRequest  data_stores=motohawk_sfun_data_def_data_stores  struct_instances=motohawk_sfun_data_def_struct_instances  vardecs=motohawk_sfun_data_def_vardecs
  motohawk_data_read1 : MotoHawk_lib/Data Storage Blocks/motohawk_data_read  source=Lookup By Name  structure=Scalar  operation=Read scalar from location by index  sz_vec=4  sz_row=2  sz_col=3  typ=double  nam='ETC_ShutdownLoAdaptError'  checkNull=on  struct_inst_name='Struct1'  struct_nam='MyStruct'
  motohawk_data_write1 : MotoHawk_lib/Data Storage Blocks/motohawk_data_write  source=Lookup By Name  structure=Scalar  operation=Write scalar into location by index  sz_vec=-1  sz_row=3  sz_col=2  typ=boolean  nam='TPSAdaptLoRequest'  checkNull=on  write_read_only=off  struct_inst_name='Struct1'  struct_name='MyStruct'
  motohawk_probe2 : MotoHawk_lib/Calibration & Probing Blocks/motohawk_probe  nam='ETC_ShutdownSetpointMode'  show_more=on  name_source=Use Parameter  read_level=1  view_as=Number  enum_struct={'Disabled', 'Enabled'}  vector_style=Wide Row  use_help_units=on  help='Shutdown mode for ETC setpoint. 0=Passthrough, 1=LoAdapt, 2=SpringTest.'  units=''  use_header_enum=off  row_header_enum={}  col_header_enum={}  use_precision=off  precision=''  gain=1  offset=0  exp=1  use_mototune_group=on  mototune_group=motohawk_vardec_path(gcb)
  wires:
  ETC Setpoint Mode/1 -> ShutDownAdaptMode/1, motohawk_probe2/1
  ShutDownAdaptMode/1 -> Logical Operator/1
  ETC Error/1 -> Relational Operator4/1
  Relational Operator4/1 -> Logical Operator/2
  Logical Operator/1 -> motohawk_data_write1/1
  motohawk_data_read1/1 -> Add1/2
  Constant1/1 -> Add1/1
  Add1/1 -> Relational Operator4/2
